simulink model "CartModelling"  (R2021a)
settings: Solver=ode1  StartTime=0.0  StopTime=30  FixedStep=0.002  RelTol=1e-3
undefined symbols (not defined in the file or in its folder): B_c
settings Model: Creator=User  LastModifiedBy=User
settings SolverCC: AutoInsertRateTranBlk=on

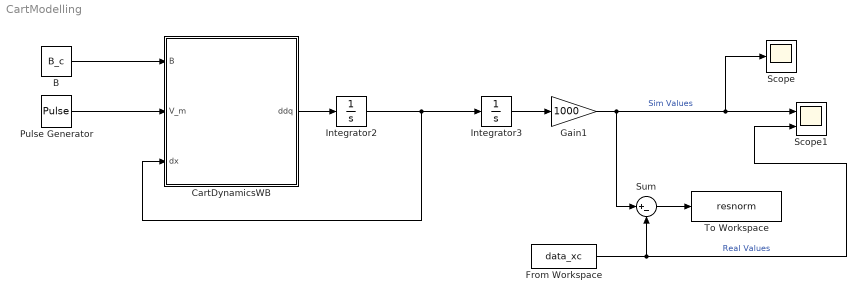
== system CartModelling ==
  B : Constant  Value=B_c
  CartDynamicsWB : MATLAB Function  TreatAsAtomicUnit=on
  From Workspace : FromWorkspace  VariableName=data_xc  OutDataTypeStr=double
  Gain1 : Gain  Gain=1000
  Integrator2 : Integrator
  Integrator3 : Integrator
  Pulse Generator : DiscretePulseGenerator  PulseType=Time based  Amplitude=4  Period=100  PulseWidth=0.1  PhaseDelay=2
  Scope : Scope
  Scope1 : Scope  NumInputPorts=2
  Sum : Sum  Inputs=|+-
  To Workspace : ToWorkspace  VariableName=resnorm  SaveFormat=Timeseries  SampleTime=-1
  wires:
  Pulse Generator/1 -> CartDynamicsWB/2(V_m)
  CartDynamicsWB/1(ddq) -> Integrator2/1
  Integrator2/1 -> CartDynamicsWB/3(dx), Integrator3/1
  Integrator3/1 -> Gain1/1
  Gain1/1 -> Scope/1, Scope1/1, Sum/1  "Sim Values"
  B/1 -> CartDynamicsWB/1(B)
  Sum/1 -> To Workspace/1
  From Workspace/1 -> Scope1/2, Sum/2  "Real Values"

== matlab function CartModelling/CartDynamicsWB ==
  data: B input; ddq output; V_m input; dx input
function ddq = CartDynamicsWB(B,V_m,dx)
%#codegen

%    This function was generated by the Symbolic Math Toolbox version 8.7.
%    07-Sep-2022 11:10:39

R_m = 2.6; 
k_t = 0.00767;
n_m = 1;
k_m = 0.00767;
K_g = 3.71;
n_g = 1;
r_mp = 6.35*10^(-3);

m_c = 0.57;

ddq = -(B.*dx-(K_g.*k_t.*n_g.*n_m.*1.0./r_mp.^2.*(V_m.*r_mp-K_g.*dx.*k_m))./R_m)./m_c;
